simulink model "newtonCannonSim"  (R2024a)
settings: Solver=ode4  StartTime=0.0  StopTime=10000  FixedStep=5  RelTol=1e-3
values from neighbouring files (symbols this model uses):
  G = 6.6743e-11    [projMotion.m]
  M = 5.97219e24    (= 5.97219e+24)    [projMotion.m]
  m = 1    [projMotion.m]
  R = 6371000    [projMotion.m]
  startHeight = .155*R    (= 987505)    [projMotion.m]
  v0 = i    [projMotion.m]
settings Model: Creator=ojaroker  LastModifiedBy=ojaroker
settings OptimizationCC: DefaultParameterBehavior=Inlined  UseDivisionForNetSlopeComputation=on  GainParamInheritBuiltInType=on  UseFloatMulNetSlope=on  InlineInvariantSignals=on  PassReuseOutputArgsAs=Individual arguments  ZeroExternalMemoryAtStartup=off  ZeroInternalMemoryAtStartup=off  NoFixptDivByZeroProtection=on  EfficientFloat2IntCast=on  LifeSpan=1  OptimizeBlockOrder=speed  DifferentSizesBufferReuse=on  EfficientTunableParamExpr=on
settings DebuggingCC: ParameterTunabilityLossMsg=error
settings HardwareCC: ProdLongLongMode=on  TargetBitPerLong=64  TargetBitPerPointer=64  TargetBitPerSizeT=64  TargetBitPerPtrDiffT=64  TargetLongLongMode=on  TargetIntDivRoundTo=Zero  TargetEndianess=LittleEndian  TargetWordSize=64  TargetHWDeviceType=MATLAB Host  ProdEqTarget=off
settings SFSimCC: MATLABDynamicMemAlloc=off
settings RTWCC: Description=Embedded Coder  SystemTargetFile=ert.tlc  GenCodeOnly=on  TemplateMakefile=ert_default_tmf  TargetLang=C++  GPUComputeCapability=3.5
settings CodeAppCC: ForceParamTrailComments=on  IgnoreCustomStorageClasses=off  OperatorAnnotations=on  SimulinkDataObjDesc=on  SFDataObjDesc=on  CustomSymbolStrGlobalVar=rt$N$M  CustomSymbolStrType=$N$M  CustomSymbolStrFcn=$N$M$F  CustomSymbolStrMacro=$N$M  InsertBlockDesc=on
settings ERTTargetCC: TargetLangStandard=C++11 (ISO)  GenerateSampleERTMain=on  IncludeMdlTerminateFcn=off  CombineSignalStateStructs=on  SupportAbsoluteTime=off  CodeInterfacePackaging=C++ class  SupportComplex=off  SupportContinuousTime=on  InlinedParameterPlacement=NonHierarchical  RootIOFormat=Structure reference  ERTCustomFileTemplate=example_file_process.tlc  ERTFilePackagingFormat=CompactWithDataFile

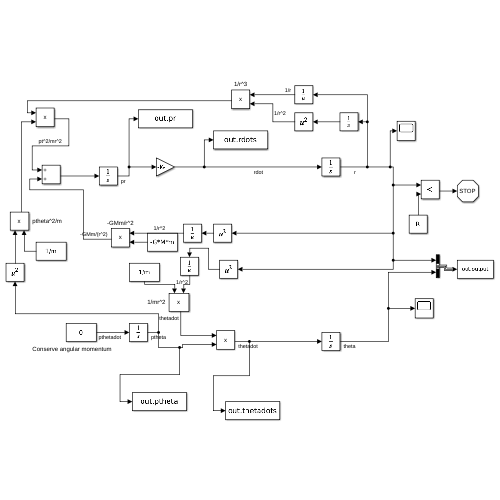
[thumbnail: Simulink's stored preview of the top-level diagram]
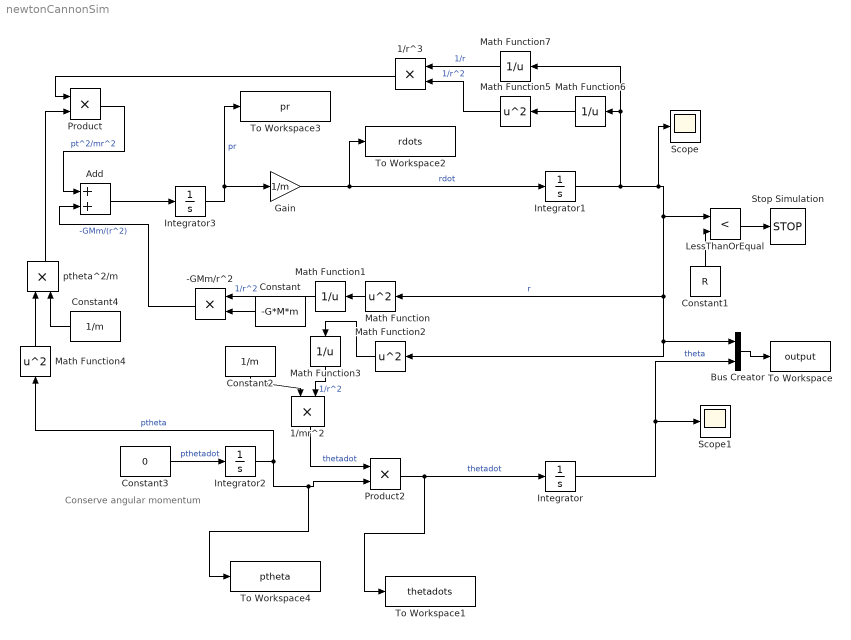
== system newtonCannonSim ==
  note: Conserve angular momentum
  -GMm/r^2 : Product
  1/mr^2 : Product
  1/r^3 : Product
  Add : Sum
  Bus Creator : BusCreator  Inputs=2
  Constant : Constant  Value=-G*M*m
  Constant1 : Constant  Value=R
  Constant2 : Constant  Value=1/m
  Constant3 : Constant  Value=0
  Constant4 : Constant  Value=1/m
  Gain : Gain  Gain=1/m
  Integrator : Integrator  InitialCondition=pi/2
  Integrator1 : Integrator  InitialCondition=R+startHeight
  Integrator2 : Integrator  InitialCondition=(R+startHeight)*v0*m
  Integrator3 : Integrator
  LessThanOrEqual : RelationalOperator  Operator=<  OutDataTypeStr=boolean  RndMeth=Simplest  InputSameDT=off
  Math Function{,2,4..5} (4 alike) : Math  Operator=square
  Math Function{1,3,6..7} (4 alike) : Math  Operator=reciprocal
  Product : Product
  Product2 : Product
  Scope : Scope
  Scope1 : Scope
  Stop Simulation : Stop
  To Workspace : ToWorkspace  VariableName=output  SampleTime=-1
  To Workspace1 : ToWorkspace  VariableName=thetadots  SampleTime=-1
  To Workspace2 : ToWorkspace  VariableName=rdots  SampleTime=-1
  To Workspace3 : ToWorkspace  VariableName=pr  SampleTime=-1
  To Workspace4 : ToWorkspace  VariableName=ptheta  SampleTime=-1
  ptheta^2/m : Product
  wires:
  Integrator1/1 -> Scope/1, LessThanOrEqual/1, Math Function/1, Bus Creator/1, Math Function2/1, Math Function7/1, Math Function6/1  "r"
  Gain/1 -> To Workspace2/1, Integrator1/1  "rdot"
  Math Function/1 -> Math Function1/1
  Constant/1 -> -GMm/r^2/2
  Math Function1/1 -> -GMm/r^2/1  "1/r^2"
  LessThanOrEqual/1 -> Stop Simulation/1
  Constant1/1 -> LessThanOrEqual/2
  Integrator3/1 -> To Workspace3/1, Gain/1  "pr"
  Math Function2/1 -> Math Function3/1
  Math Function3/1 -> 1/mr^2/2  "1/r^2"
  Constant2/1 -> 1/mr^2/1
  1/mr^2/1 -> Product2/1  "thetadot"
  Integrator2/1 -> To Workspace4/1, Product2/2, Math Function4/1  "ptheta"
  Constant3/1 -> Integrator2/1  "pthetadot"
  Integrator/1 -> Scope1/1, Bus Creator/2  "theta"
  Bus Creator/1 -> To Workspace/1
  Product2/1 -> Integrator/1, To Workspace1/1  "thetadot"
  -GMm/r^2/1 -> Add/2  "-GMm/(r^2)"
  Math Function4/1 -> ptheta^2/m/1
  Math Function6/1 -> Math Function5/1
  Math Function5/1 -> 1/r^3/2  "1/r^2"
  Math Function7/1 -> 1/r^3/1  "1/r"
  Constant4/1 -> ptheta^2/m/2
  ptheta^2/m/1 -> Product/2
  1/r^3/1 -> Product/1
  Product/1 -> Add/1  "pt^2/mr^2"
  Add/1 -> Integrator3/1
